simulink model "func_modelo_iter2"  (R2018a)
settings: Solver=VariableStepAuto  StartTime=0.0  StopTime=5000  RelTol=1e-3
libraries: simulink x6
settings Model: Creator=catalina  LastModifiedBy=catalina

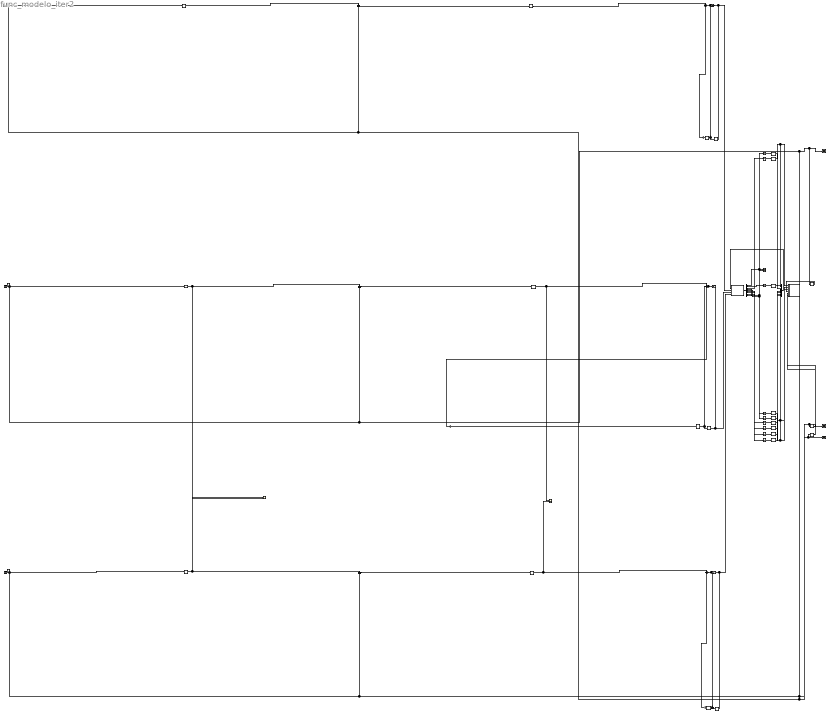
== system func_modelo_iter2 ==
  Demux : Demux  Outputs=9
  Gain : Gain
  Gain1 : Gain
  Gain2 : Gain
  Integrator : Integrator  InitialCondition=63/2
  Integrator{1,3..8} (7 alike) : Integrator
  Integrator2 : Integrator  InitialCondition=2200
  MATLAB Function : MATLAB Function  TreatAsAtomicUnit=on
  MATLAB Function1 : MATLAB Function  TreatAsAtomicUnit=on
  PID Controller1 : simulink/Continuous/PID Controller  Controller=PID  TimeDomain=Continuous-time  SampleTime=-1  IntegratorMethod=Forward Euler  FilterMethod=Forward Euler  Form=Parallel  UseFilter=on  ControllerParametersSource=internal  P=0  I=0  D=-30.7973  N=3.3865  InitialConditionSource=internal  InitialConditionForIntegrator=0  InitialConditionForFilter=0  ExternalReset=none  LimitOutput=off  UpperSaturationLimit=inf  LowerSaturationLimit=-inf  LinearizeAsGain=on  AntiWindupMode=none  Kb=1  TrackingMode=off  Kt=1  PParamMin=[]  PParamMax=[]  IParamMin=[]  IParamMax=[]  DParamMin=[]  DParamMax=[]  NParamMin=[]  NParamMax=[]  KbParamMin=[]  KbParamMax=[]  KtParamMin=[]  KtParamMax=[]  POutMin=[]  POutMax=[]  IOutMin=[]  IOutMax=[]  DOutMin=[]  DOutMax=[]  NOutMin=[]  NOutMax=[]  KbOutMin=[]  KbOutMax=[]  KtOutMin=[]  KtOutMax=[]  IntegratorOutMin=[]  IntegratorOutMax=[]  FilterOutMin=[]  FilterOutMax=[]  SumOutMin=[]  SumOutMax=[]  SumI1OutMin=[]  SumI1OutMax=[]  SumI2OutMin=[]  SumI2OutMax=[]  SumI3OutMin=[]  SumI3OutMax=[]  SumDOutMin=[]  SumDOutMax=[]  SaturationOutMin=[]  SaturationOutMax=[]  IntegratorContinuousStateAttributes=''  IntegratorStateMustResolveToSignalObject=off  IntegratorRTWStateStorageClass=Auto  FilterContinuousStateAttributes=''  FilterStateMustResolveToSignalObject=off  FilterRTWStateStorageClass=Auto  DifferentiatorICPrevScaledInput=0  DifferentiatorOutMin=[]  DifferentiatorOutMax=[]  FilterDiffOutCoefMin=[]  FilterDiffOutCoefMax=[]  SumDenOutMin=[]  SumDenOutMax=[]  SumNumOutMin=[]  SumNumOutMax=[]  ReciprocalOutMin=[]  ReciprocalOutMax=[]  DivideOutMin=[]  DivideOutMax=[]  TunerSelectOption=Transfer Function Based (PID Tuner App)
  PID Controller2 : simulink/Continuous/PID Controller  Controller=PID  TimeDomain=Continuous-time  SampleTime=-1  IntegratorMethod=Forward Euler  FilterMethod=Forward Euler  Form=Parallel  UseFilter=on  ControllerParametersSource=internal  P=0  I=12.3301  D=0  N=100  InitialConditionSource=internal  InitialConditionForIntegrator=0  InitialConditionForFilter=0  ExternalReset=none  LimitOutput=off  UpperSaturationLimit=inf  LowerSaturationLimit=-inf  LinearizeAsGain=on  AntiWindupMode=none  Kb=1  TrackingMode=off  Kt=1  PParamMin=[]  PParamMax=[]  IParamMin=[]  IParamMax=[]  DParamMin=[]  DParamMax=[]  NParamMin=[]  NParamMax=[]  KbParamMin=[]  KbParamMax=[]  KtParamMin=[]  KtParamMax=[]  POutMin=[]  POutMax=[]  IOutMin=[]  IOutMax=[]  DOutMin=[]  DOutMax=[]  NOutMin=[]  NOutMax=[]  KbOutMin=[]  KbOutMax=[]  KtOutMin=[]  KtOutMax=[]  IntegratorOutMin=[]  IntegratorOutMax=[]  FilterOutMin=[]  FilterOutMax=[]  SumOutMin=[]  SumOutMax=[]  SumI1OutMin=[]  SumI1OutMax=[]  SumI2OutMin=[]  SumI2OutMax=[]  SumI3OutMin=[]  SumI3OutMax=[]  SumDOutMin=[]  SumDOutMax=[]  SaturationOutMin=[]  SaturationOutMax=[]  IntegratorContinuousStateAttributes=''  IntegratorStateMustResolveToSignalObject=off  IntegratorRTWStateStorageClass=Auto  FilterContinuousStateAttributes=''  FilterStateMustResolveToSignalObject=off  FilterRTWStateStorageClass=Auto  DifferentiatorICPrevScaledInput=0  DifferentiatorOutMin=[]  DifferentiatorOutMax=[]  FilterDiffOutCoefMin=[]  FilterDiffOutCoefMax=[]  SumDenOutMin=[]  SumDenOutMax=[]  SumNumOutMin=[]  SumNumOutMax=[]  ReciprocalOutMin=[]  ReciprocalOutMax=[]  DivideOutMin=[]  DivideOutMax=[]  TunerSelectOption=Transfer Function Based (PID Tuner App)
  PID Controller3 : simulink/Continuous/PID Controller  Controller=PID  TimeDomain=Continuous-time  SampleTime=-1  IntegratorMethod=Forward Euler  FilterMethod=Forward Euler  Form=Parallel  UseFilter=on  ControllerParametersSource=internal  P=0  I=75.7322  D=0  N=100  InitialConditionSource=internal  InitialConditionForIntegrator=0  InitialConditionForFilter=0  ExternalReset=none  LimitOutput=off  UpperSaturationLimit=inf  LowerSaturationLimit=-inf  LinearizeAsGain=on  AntiWindupMode=none  Kb=1  TrackingMode=off  Kt=1  PParamMin=[]  PParamMax=[]  IParamMin=[]  IParamMax=[]  DParamMin=[]  DParamMax=[]  NParamMin=[]  NParamMax=[]  KbParamMin=[]  KbParamMax=[]  KtParamMin=[]  KtParamMax=[]  POutMin=[]  POutMax=[]  IOutMin=[]  IOutMax=[]  DOutMin=[]  DOutMax=[]  NOutMin=[]  NOutMax=[]  KbOutMin=[]  KbOutMax=[]  KtOutMin=[]  KtOutMax=[]  IntegratorOutMin=[]  IntegratorOutMax=[]  FilterOutMin=[]  FilterOutMax=[]  SumOutMin=[]  SumOutMax=[]  SumI1OutMin=[]  SumI1OutMax=[]  SumI2OutMin=[]  SumI2OutMax=[]  SumI3OutMin=[]  SumI3OutMax=[]  SumDOutMin=[]  SumDOutMax=[]  SaturationOutMin=[]  SaturationOutMax=[]  IntegratorContinuousStateAttributes=''  IntegratorStateMustResolveToSignalObject=off  IntegratorRTWStateStorageClass=Auto  FilterContinuousStateAttributes=''  FilterStateMustResolveToSignalObject=off  FilterRTWStateStorageClass=Auto  DifferentiatorICPrevScaledInput=0  DifferentiatorOutMin=[]  DifferentiatorOutMax=[]  FilterDiffOutCoefMin=[]  FilterDiffOutCoefMax=[]  SumDenOutMin=[]  SumDenOutMax=[]  SumNumOutMin=[]  SumNumOutMax=[]  ReciprocalOutMin=[]  ReciprocalOutMax=[]  DivideOutMin=[]  DivideOutMax=[]  TunerSelectOption=Transfer Function Based (PID Tuner App)
  PID Controller4 : simulink/Continuous/PID Controller  Controller=PID  TimeDomain=Continuous-time  SampleTime=-1  IntegratorMethod=Forward Euler  FilterMethod=Forward Euler  Form=Parallel  UseFilter=on  ControllerParametersSource=internal  P=0  I=75.7322  D=0  N=100  InitialConditionSource=internal  InitialConditionForIntegrator=0  InitialConditionForFilter=0  ExternalReset=none  LimitOutput=off  UpperSaturationLimit=inf  LowerSaturationLimit=-inf  LinearizeAsGain=on  AntiWindupMode=none  Kb=1  TrackingMode=off  Kt=1  PParamMin=[]  PParamMax=[]  IParamMin=[]  IParamMax=[]  DParamMin=[]  DParamMax=[]  NParamMin=[]  NParamMax=[]  KbParamMin=[]  KbParamMax=[]  KtParamMin=[]  KtParamMax=[]  POutMin=[]  POutMax=[]  IOutMin=[]  IOutMax=[]  DOutMin=[]  DOutMax=[]  NOutMin=[]  NOutMax=[]  KbOutMin=[]  KbOutMax=[]  KtOutMin=[]  KtOutMax=[]  IntegratorOutMin=[]  IntegratorOutMax=[]  FilterOutMin=[]  FilterOutMax=[]  SumOutMin=[]  SumOutMax=[]  SumI1OutMin=[]  SumI1OutMax=[]  SumI2OutMin=[]  SumI2OutMax=[]  SumI3OutMin=[]  SumI3OutMax=[]  SumDOutMin=[]  SumDOutMax=[]  SaturationOutMin=[]  SaturationOutMax=[]  IntegratorContinuousStateAttributes=''  IntegratorStateMustResolveToSignalObject=off  IntegratorRTWStateStorageClass=Auto  FilterContinuousStateAttributes=''  FilterStateMustResolveToSignalObject=off  FilterRTWStateStorageClass=Auto  DifferentiatorICPrevScaledInput=0  DifferentiatorOutMin=[]  DifferentiatorOutMax=[]  FilterDiffOutCoefMin=[]  FilterDiffOutCoefMax=[]  SumDenOutMin=[]  SumDenOutMax=[]  SumNumOutMin=[]  SumNumOutMax=[]  ReciprocalOutMin=[]  ReciprocalOutMax=[]  DivideOutMin=[]  DivideOutMax=[]  TunerSelectOption=Transfer Function Based (PID Tuner App)
  PID Controller5 : simulink/Continuous/PID Controller  Controller=PID  TimeDomain=Continuous-time  SampleTime=-1  IntegratorMethod=Forward Euler  FilterMethod=Forward Euler  Form=Parallel  UseFilter=on  ControllerParametersSource=internal  P=0  I=12.3301  D=0  N=100  InitialConditionSource=internal  InitialConditionForIntegrator=0  InitialConditionForFilter=0  ExternalReset=none  LimitOutput=off  UpperSaturationLimit=inf  LowerSaturationLimit=-inf  LinearizeAsGain=on  AntiWindupMode=none  Kb=1  TrackingMode=off  Kt=1  PParamMin=[]  PParamMax=[]  IParamMin=[]  IParamMax=[]  DParamMin=[]  DParamMax=[]  NParamMin=[]  NParamMax=[]  KbParamMin=[]  KbParamMax=[]  KtParamMin=[]  KtParamMax=[]  POutMin=[]  POutMax=[]  IOutMin=[]  IOutMax=[]  DOutMin=[]  DOutMax=[]  NOutMin=[]  NOutMax=[]  KbOutMin=[]  KbOutMax=[]  KtOutMin=[]  KtOutMax=[]  IntegratorOutMin=[]  IntegratorOutMax=[]  FilterOutMin=[]  FilterOutMax=[]  SumOutMin=[]  SumOutMax=[]  SumI1OutMin=[]  SumI1OutMax=[]  SumI2OutMin=[]  SumI2OutMax=[]  SumI3OutMin=[]  SumI3OutMax=[]  SumDOutMin=[]  SumDOutMax=[]  SaturationOutMin=[]  SaturationOutMax=[]  IntegratorContinuousStateAttributes=''  IntegratorStateMustResolveToSignalObject=off  IntegratorRTWStateStorageClass=Auto  FilterContinuousStateAttributes=''  FilterStateMustResolveToSignalObject=off  FilterRTWStateStorageClass=Auto  DifferentiatorICPrevScaledInput=0  DifferentiatorOutMin=[]  DifferentiatorOutMax=[]  FilterDiffOutCoefMin=[]  FilterDiffOutCoefMax=[]  SumDenOutMin=[]  SumDenOutMax=[]  SumNumOutMin=[]  SumNumOutMax=[]  ReciprocalOutMin=[]  ReciprocalOutMax=[]  DivideOutMin=[]  DivideOutMax=[]  TunerSelectOption=Transfer Function Based (PID Tuner App)
  PID Controller6 : simulink/Continuous/PID Controller  Controller=PID  TimeDomain=Continuous-time  SampleTime=-1  IntegratorMethod=Forward Euler  FilterMethod=Forward Euler  Form=Parallel  UseFilter=on  ControllerParametersSource=internal  P=-17.7709  I=0  D=-3.5395  N=3  InitialConditionSource=internal  InitialConditionForIntegrator=0  InitialConditionForFilter=0  ExternalReset=none  LimitOutput=off  UpperSaturationLimit=inf  LowerSaturationLimit=-inf  LinearizeAsGain=on  AntiWindupMode=none  Kb=1  TrackingMode=off  Kt=1  PParamMin=[]  PParamMax=[]  IParamMin=[]  IParamMax=[]  DParamMin=[]  DParamMax=[]  NParamMin=[]  NParamMax=[]  KbParamMin=[]  KbParamMax=[]  KtParamMin=[]  KtParamMax=[]  POutMin=[]  POutMax=[]  IOutMin=[]  IOutMax=[]  DOutMin=[]  DOutMax=[]  NOutMin=[]  NOutMax=[]  KbOutMin=[]  KbOutMax=[]  KtOutMin=[]  KtOutMax=[]  IntegratorOutMin=[]  IntegratorOutMax=[]  FilterOutMin=[]  FilterOutMax=[]  SumOutMin=[]  SumOutMax=[]  SumI1OutMin=[]  SumI1OutMax=[]  SumI2OutMin=[]  SumI2OutMax=[]  SumI3OutMin=[]  SumI3OutMax=[]  SumDOutMin=[]  SumDOutMax=[]  SaturationOutMin=[]  SaturationOutMax=[]  IntegratorContinuousStateAttributes=''  IntegratorStateMustResolveToSignalObject=off  IntegratorRTWStateStorageClass=Auto  FilterContinuousStateAttributes=''  FilterStateMustResolveToSignalObject=off  FilterRTWStateStorageClass=Auto  DifferentiatorICPrevScaledInput=0  DifferentiatorOutMin=[]  DifferentiatorOutMax=[]  FilterDiffOutCoefMin=[]  FilterDiffOutCoefMax=[]  SumDenOutMin=[]  SumDenOutMax=[]  SumNumOutMin=[]  SumNumOutMax=[]  ReciprocalOutMin=[]  ReciprocalOutMax=[]  DivideOutMin=[]  DivideOutMax=[]  TunerSelectOption=Transfer Function Based (PID Tuner App)
  Saturation : Saturate  UpperLimit=10  LowerLimit=0
  Saturation1 : Saturate  UpperLimit=0.3*pi/180  LowerLimit=-0.3*pi/180
  Saturation2 : Saturate  UpperLimit=0.3*pi/180  LowerLimit=-0.3*pi/180
  Scope : Scope
  Scope1 : Scope
  Scope2 : Scope
  Scope3 : Scope  NumInputPorts=3
  Scope4 : Scope  NumInputPorts=2
  Scope5 : Scope  NumInputPorts=2
  Step : Step  After=10000  SampleTime=0
  Step1 : Step  After=1000  SampleTime=0
  Step2 : Step  After=1000  SampleTime=0
  Sum{,1..11} (12 alike) : Sum  Inputs=+-
  Transport Delay{,1,3..11} (11 alike) : TransportDelay
  Transport Delay{2,12..17} (7 alike) : TransportDelay  InitialOutput=1
  Vector Concatenate : Concatenate  NumInputs=9
  wires:
  Integrator/1 -> Transport Delay/1
  Integrator1/1 -> Transport Delay1/1
  Integrator2/1 -> Transport Delay2/1
  Integrator3/1 -> Transport Delay3/1
  Integrator4/1 -> Transport Delay4/1
  Integrator5/1 -> Transport Delay5/1
  Integrator6/1 -> Transport Delay6/1
  Integrator7/1 -> Transport Delay7/1
  Integrator8/1 -> Transport Delay8/1
  MATLAB Function/1(xprima) -> Demux/1
  Demux/1 -> Scope3/1, Integrator/1
  Demux/2 -> Integrator1/1
  Demux/3 -> Integrator2/1
  Demux/4 -> Scope3/2, Integrator3/1
  Demux/5 -> Scope3/3, Integrator4/1
  Demux/6 -> Integrator5/1
  Demux/7 -> Integrator6/1
  Demux/8 -> Integrator7/1
  Demux/9 -> Integrator8/1
  Transport Delay/1 -> Vector Concatenate/1
  Transport Delay1/1 -> MATLAB Function1/1(vel), Vector Concatenate/2
  Transport Delay2/1 -> Vector Concatenate/3
  Transport Delay3/1 -> MATLAB Function1/2(phi), Vector Concatenate/4
  Transport Delay4/1 -> MATLAB Function1/3(theta), Vector Concatenate/5
  Transport Delay5/1 -> Vector Concatenate/6
  Transport Delay6/1 -> Vector Concatenate/7
  Transport Delay7/1 -> Vector Concatenate/8
  Transport Delay8/1 -> Vector Concatenate/9
  Vector Concatenate/1 -> MATLAB Function/2(x)
  MATLAB Function1/1(x) -> Transport Delay9/1, Scope/1, Sum4/2, Sum5/2
  MATLAB Function1/3(h) -> Scope2/1, Transport Delay11/1, Sum/2, Sum1/2
  Transport Delay9/1 -> MATLAB Function1/4(xant)
  Transport Delay10/1 -> MATLAB Function1/5(yant)
  Transport Delay11/1 -> MATLAB Function1/6(zant)
  Step/1 -> Sum/1
  Sum2/1 -> Sum3/1, Saturation/1
  Saturation/1 -> Transport Delay12/1, MATLAB Function/3(ut)
  Gain/1 -> Sum2/2
  Gain1/1 -> Sum6/2
  Sum6/1 -> Saturation1/1, Sum7/1
  Saturation1/1 -> MATLAB Function/4(ux), Transport Delay13/1
  Step1/1 -> Sum4/1
  Saturation2/1 -> Transport Delay14/1, MATLAB Function/5(uy)
  MATLAB Function1/2(y) -> Scope1/1, Transport Delay10/1, Sum8/2, Sum9/2
  Sum10/1 -> Sum11/1, Saturation2/1
  Gain2/1 -> Sum10/2
  Step2/1 -> Sum8/1
  Transport Delay12/1 -> Sum3/2
  Transport Delay13/1 -> Sum7/2
  Transport Delay14/1 -> Sum11/2
  Transport Delay15/1 -> Gain1/1
  Sum7/1 -> Transport Delay15/1
  Transport Delay16/1 -> Gain2/1
  Sum11/1 -> Transport Delay16/1
  Transport Delay17/1 -> Gain/1
  Sum3/1 -> Transport Delay17/1
  PID Controller1/1 -> Sum1/1
  Sum/1 -> PID Controller1/1
  PID Controller6/1 -> Sum2/1
  Sum1/1 -> PID Controller6/1
  Sum9/1 -> PID Controller5/1
  PID Controller4/1 -> Scope4/2, Sum9/1
  Sum8/1 -> PID Controller4/1
  Sum5/1 -> PID Controller2/1
  PID Controller3/1 -> Scope4/1, Sum5/1
  Sum4/1 -> PID Controller3/1
  PID Controller2/1 -> Scope5/1, Sum6/1
  PID Controller5/1 -> Scope5/2, Sum10/1

== matlab function func_modelo_iter2/MATLAB Function1 ==
  data: x output; vel input; y output; phi input; theta input; xant input; yant input; zant input; h output
function [x, y, h]=cartesianas(vel, phi, theta, xant,yant, zant)
Ts = 0.1;

x = xant + vel*cos(phi)*cos(theta)*Ts;
y = yant + vel*cos(phi)*sin(theta)*Ts;
h = zant + vel*sin(phi)*Ts;

% if x < 0
%     x = 0;
% end
% 
% if y < 0
%     y = 0;
% end

if h < 0
    h = 0;
end

== matlab function func_modelo_iter2/MATLAB Function ==
  data: t input; xprima output; x input; ut input; ux input; uy input
function xprima=cohete_modelov2(t,x,ut,ux,uy)
xprima = zeros(1,9);
g0 = 9.8065;  % gravedad (se asume constante en altura)
ro0= 0.1; % coef resistencia superficie terrestre
ve=5000; % velocidad de escape de gases
Ac=7.5; % area transversal para calculo de roce con aire
Mmin=100; % masa del cohete sin combustible

%Ruido
mu=0;
sigma=0.5*pi/180;

% maximos para tobera
utMax=10; % maximo empuje longitudinal
uxMax=0.3*pi/180;  % maxima inclinacion tobera en eje x del cohete
uyMax=0.3*pi/180;  % maxima inclinacion tobera en eje y del cohete

if x(3)<Mmin   % se acabo el combustible
    ut=0;
end

L=63; % largo cohete
Ir=x(3)*L^2/12; % momento de inercia rotacional cohete

% FUERZAS MAXIMAS
if ut>utMax, ut=utMax; end;
if ut<0, ut=0; end;


if ux>uxMax, ux=uxMax; end;
if ux<-uxMax, ux=-uxMax; end;
if uy>uyMax, uy=uyMax; end;
if uy<-uyMax, uy=-uyMax; end;


% ECUACIONES DIFERENCIALES SIMPLIFICADAS
% g=g0*(Rs/(Rs+x(1))); % gravedad
Ftob=ut*ve; % fuerza tobera empuje, thrust
Fux=Ftob*sin(x(8)); % componente de fuerza tobera transversal X
Fuy=Ftob*sin(x(9)); % componente de fuerza tobera transversal Y
Fp=sqrt((Ftob)^2-Fux^2-Fuy^2); % fuerza empuje vertical
ro=ro0*((1 - (x(1)/20000)^2)>0)*(1 - (x(1)/20000)^2); % roce aire



xprima(1)=x(2); % dh/dt
xprima(2)=(Fp - ro*Ac*sign(x(2))*abs(x(2))^(3/2)- x(3)*g0*sin(x(4)))/x(3); % dh^2/dt^2
xprima(3)=-ut; % dM/dT
xprima(4)=x(6); % d_phi/dt
xprima(5)=x(7);%+normrnd(mu,sigma); % d_theta/dt
xprima(6)=(L/2)*(Fux-1*g0*cos(x(4))-1500*x(6))/Ir;  % d^2_phi/dt^2
xprima(7)=(L/2)*(Fuy-1500*x(7))/Ir;  % d^2_theta/dt^2
xprima(8) = (ux-x(8))/2;
xprima(9) = (uy-x(9))/2;

% [x(8),xprima(8)]

% xprima=xprima';
